simulink model "prelab"  (R2022a)
settings: Solver=VariableStepAuto  StartTime=0.0  StopTime=10  RelTol=1e-3
undefined symbols (not defined in the file): A1, B1, F1
settings Model: Creator=varunsampat  LastModifiedBy=user
settings DebuggingCC: UnconnectedInputMsg=warning  UnconnectedOutputMsg=warning  UnconnectedLineMsg=warning
settings RTWCC: DLArmComputeVersion=19.05

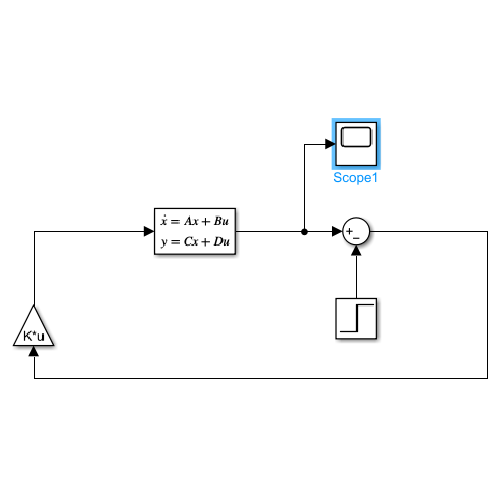
[thumbnail: Simulink's stored preview of the top-level diagram]
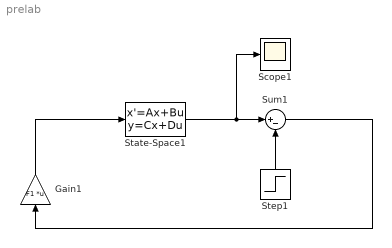
== system prelab ==
  Gain1 : Gain  Gain=F1  Multiplication=Matrix(K*u)
  Scope1 : Scope
  State-Space1 : StateSpace  A=A1  B=B1  C=eye(4)  D=zeros(4,1)  InitialCondition=[0;0;0;0]
  Step1 : Step  Before=[0; 0; 0; 0]  After=[1; 0; 0; 0]  SampleTime=0
  Sum1 : Sum  Inputs=|+-
  wires:
  Gain1/1 -> State-Space1/1
  State-Space1/1 -> Scope1/1, Sum1/1
  Step1/1 -> Sum1/2
  Sum1/1 -> Gain1/1
